simulink model "CC"  (R2018b)
settings: Solver=VariableStepAuto  StartTime=0.0  StopTime=5  MaxStep=1e-4  RelTol=1e-3
values from neighbouring files (symbols this model uses):
  B = 0.1    [sys1.m]
  J = 0.1    [sys1.m]
  Ke = 0.1    [sys1.m]
  Ki = wcc*Ra    (= 628.318530718)    [sys1.m]
  Kp = wcc*La    (= 6.28318530718)    [sys1.m]
  Kps = wsc*J    (= 31.4159265359)    [sys1.m]
  Kss = wsc*B    (= 31.4159265359)    [sys1.m]
  Kt = 0.1    [sys1.m]
  La = 1e-3    (= 0.001)    [sys1.m]
  Ra = 0.1    [sys1.m]
settings Model: Creator=kitty  LastModifiedBy=kitty

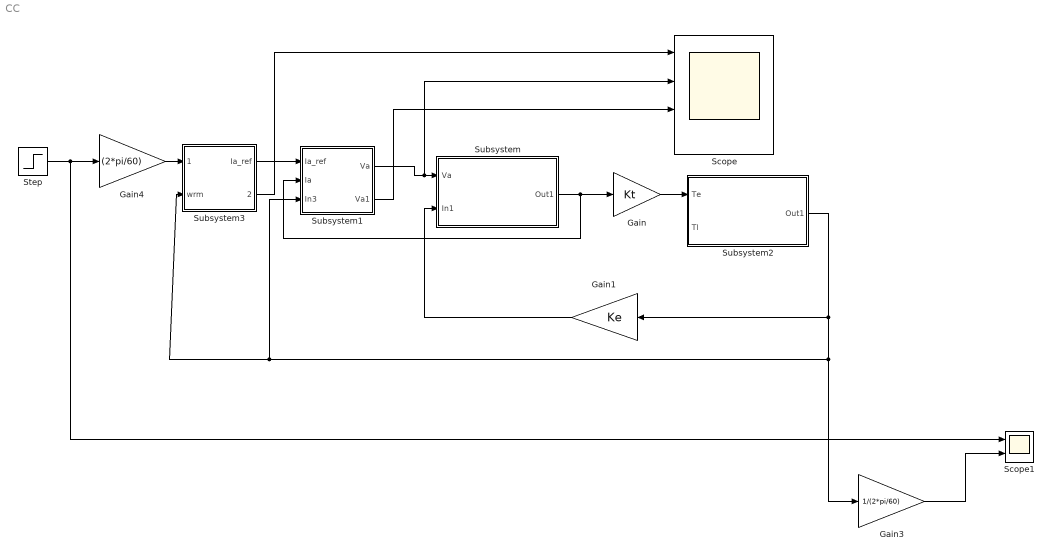
== system CC ==
  Gain : Gain  Gain=Kt
  Gain1 : Gain  Gain=Ke
  Gain3 : Gain  Gain=1/(2*pi/60)
  Gain4 : Gain  Gain=(2*pi/60)
  Scope : Scope  NumInputPorts=4
  Scope1 : Scope  NumInputPorts=2
  Step : Step  Time=0.1  After=2000  SampleTime=0
  Subsystem : Subsystem
  Subsystem1 : Subsystem
  Subsystem2 : Subsystem
  Subsystem3 : Subsystem
  wires:
  Subsystem1/1(Va) -> Scope/2, Subsystem/1(Va)
  Subsystem/1(Out1) -> Subsystem1/2(Ia), Gain/1
  Gain/1 -> Subsystem2/1(Te)
  Gain1/1 -> Subsystem/2(In1)
  Subsystem2/1(Out1) -> Gain1/1, Subsystem3/2(wrm), Subsystem1/3(In3), Gain3/1
  Subsystem3/1("Ia_ref ") -> Subsystem1/1(Ia_ref)
  Step/1 -> Scope1/1, Gain4/1
  Gain3/1 -> Scope1/2
  Gain4/1 -> Subsystem3/1(wrm_ref)
  Subsystem3/2("wrm_err ") -> Scope/1
  Subsystem1/2(Va1) -> Scope/3

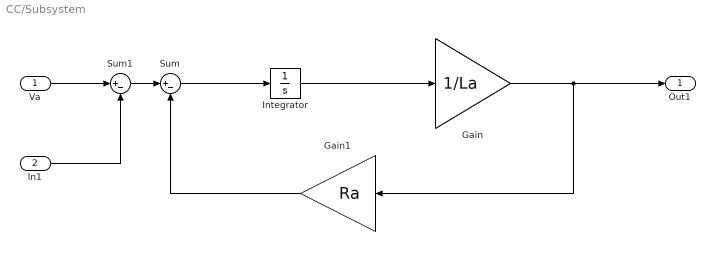
== system CC/Subsystem ==
  Va : Inport
  In1 : Inport  Port=2
  Gain : Gain  Gain=1/La
  Gain1 : Gain  Gain=Ra
  Integrator : Integrator
  Sum : Sum  Inputs=|+-
  Sum1 : Sum  Inputs=|+-
  Out1 : Outport
  wires:
  Gain/1 -> Gain1/1, Out1/1
  Integrator/1 -> Gain/1
  Gain1/1 -> Sum/2
  Sum/1 -> Integrator/1
  Va/1 -> Sum1/1
  In1/1 -> Sum1/2
  Sum1/1 -> Sum/1

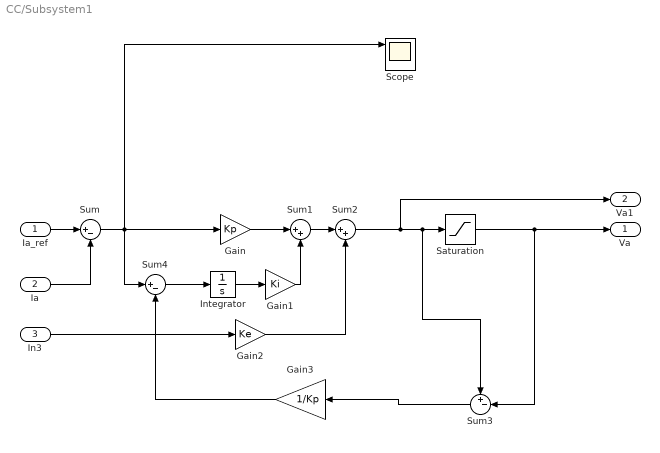
== system CC/Subsystem1 ==
  Ia_ref : Inport
  Ia : Inport  Port=2
  In3 : Inport  Port=3
  Gain : Gain  Gain=Kp
  Gain1 : Gain  Gain=Ki
  Gain2 : Gain  Gain=Ke
  Gain3 : Gain  Gain=1/Kp
  Integrator : Integrator
  Saturation : Saturate  UpperLimit=100  LowerLimit=-100
  Scope : Scope  NumInputPorts=3
  Sum : Sum  Inputs=|+-
  Sum1 : Sum  Inputs=|++
  Sum2 : Sum  Inputs=|++
  Sum3 : Sum  Inputs=+-|
  Sum4 : Sum  Inputs=|+-
  Va : Outport
  Va1 : Outport  Port=2
  wires:
  Sum/1 -> Scope/1, Sum4/1, Gain/1
  Gain/1 -> Sum1/1
  Integrator/1 -> Gain1/1
  Gain1/1 -> Sum1/2
  Ia_ref/1 -> Sum/1
  Ia/1 -> Sum/2
  In3/1 -> Gain2/1
  Gain2/1 -> Sum2/2
  Sum1/1 -> Sum2/1
  Sum2/1 -> Va1/1, Sum3/1, Saturation/1
  Saturation/1 -> Sum3/2, Va/1
  Sum3/1 -> Gain3/1
  Sum4/1 -> Integrator/1
  Gain3/1 -> Sum4/2

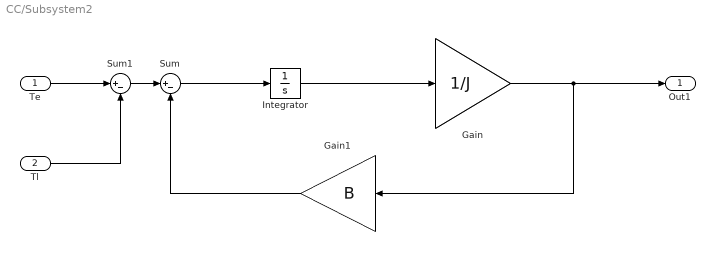
== system CC/Subsystem2 ==
  Te : Inport
  Tl : Inport  Port=2
  Gain : Gain  Gain=1/J
  Gain1 : Gain  Gain=B
  Integrator : Integrator
  Sum : Sum  Inputs=|+-
  Sum1 : Sum  Inputs=|+-
  Out1 : Outport
  wires:
  Sum1/1 -> Sum/1
  Tl/1 -> Sum1/2
  Te/1 -> Sum1/1
  Sum/1 -> Integrator/1
  Gain1/1 -> Sum/2
  Integrator/1 -> Gain/1
  Gain/1 -> Out1/1, Gain1/1

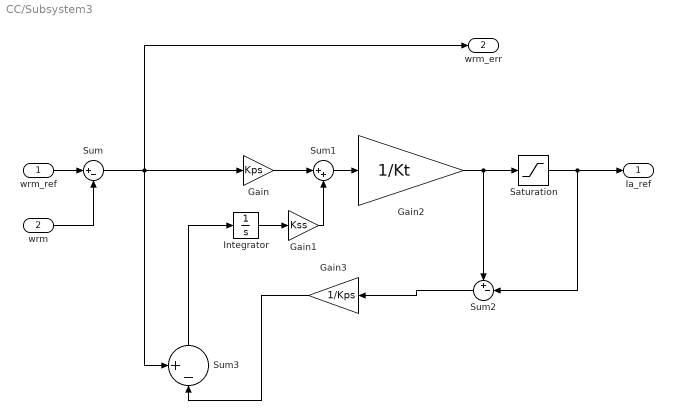
== system CC/Subsystem3 ==
  wrm_ref : Inport
  wrm : Inport  Port=2
  Gain : Gain  Gain=Kps
  Gain1 : Gain  Gain=Kss
  Gain2 : Gain  Gain=1/Kt
  Gain3 : Gain  Gain=1/Kps
  Integrator : Integrator
  Saturation : Saturate  UpperLimit=200  LowerLimit=-200
  Sum : Sum  Inputs=|+-
  Sum1 : Sum  Inputs=|++
  Sum2 : Sum  Inputs=+-|
  Sum3 : Sum  Inputs=+-|
  "Ia_ref " : Outport
  "wrm_err " : Outport  Port=2
  wires:
  Gain2/1 -> Sum2/1, Saturation/1
  Sum1/1 -> Gain2/1
  wrm/1 -> Sum/2
  wrm_ref/1 -> Sum/1
  Gain1/1 -> Sum1/2
  Integrator/1 -> Gain1/1
  Gain/1 -> Sum1/1
  Sum/1 -> Sum3/1, "wrm_err "/1, Gain/1
  Saturation/1 -> Sum2/2, "Ia_ref "/1
  Sum2/1 -> Gain3/1
  Gain3/1 -> Sum3/2
  Sum3/1 -> Integrator/1
